simulink model "Ejercicio_2"  (R2013a)
settings: Solver=ode45  StartTime=0.0  StopTime=10.0  RelTol=1e-3
values from neighbouring files (symbols this model uses):
  G1 = 1/(s+7)    [Ecuaciones3_Practica_1.m]    (also in Ecuaciones_Practica_1.m; RLC_3.m = Vl/Vi; RL_1.m = w./sqrt(w.^2+(R/L)^2))
  G2 = 1/(s^2+2*s+3)    [Ecuaciones3_Practica_1.m]    (also in Ecuaciones_Practica_1.m; RLC_3.m = Vr/Vi; RL_1.m = (R/L)./sqrt(w.^2+(R/L)^2))
  G3 = 1/(s+4)    [Ecuaciones3_Practica_1.m]    (also in Ecuaciones_Practica_1.m)
  G4 = 1/s    [Ecuaciones3_Practica_1.m]    (also in Ecuaciones_Practica_1.m)
  G5 = 5/(s+7)    [Ecuaciones3_Practica_1.m]    (also in Ecuaciones_Practica_1.m)
  G6 = 1/(s^2+5*s+10)    [Ecuaciones3_Practica_1.m]    (also in Ecuaciones_Practica_1.m)
  G7 = 3/(s+2)    [Ecuaciones3_Practica_1.m]    (also in Ecuaciones_Practica_1.m)
  G8 = 1/(s+6)    [Ecuaciones3_Practica_1.m]    (also in Ecuaciones_Practica_1.m)
undefined symbols (not defined in the file or in its folder): Rs, Ys
settings Model: Creator=LuisFernando  LastModifiedBy=LuisFernando

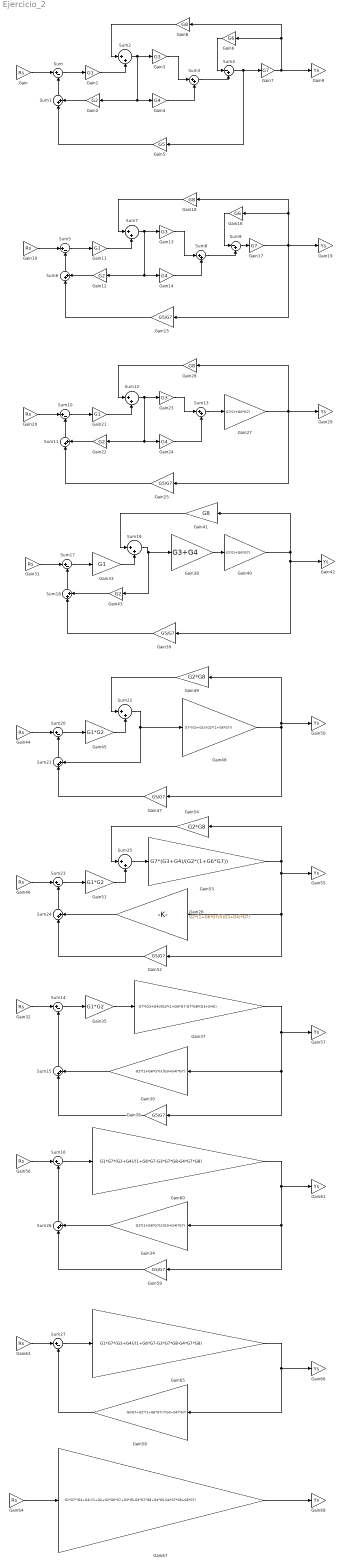
== system Ejercicio_2 ==
  Gain{,10,20,31..32,44,46,56,63..64} (10 alike) : Gain  Gain=Rs
  Gain{1,11,21,33} (4 alike) : Gain  Gain=G1
  Gain{2,12,22,43} (4 alike) : Gain  Gain=G2
  Gain13 : Gain  Gain=G3
  Gain14 : Gain  Gain=G4
  Gain{15,25,36,39,47,52,59} (7 alike) : Gain  Gain=G5/G7
  Gain16 : Gain  Gain=G6
  Gain17 : Gain  Gain=G7
  Gain{8,18,28,41} (4 alike) : Gain  Gain=G8
  Gain{9,19,29,42,50,55,57,61,66,68} (10 alike) : Gain  Gain=Ys
  Gain23 : Gain  Gain=G3
  Gain24 : Gain  Gain=G4
  Gain26 : Gain  Gain=G2*(1+G6*G7)/((G3+G4)*G7)
  Gain27 : Gain  Gain=G7/(1+G6*G7)
  Gain3 : Gain  Gain=G3
  Gain30 : Gain  Gain=G2*(1+G6*G7)/((G3+G4)*G7)
  Gain34 : Gain  Gain=G2*(1+G6*G7)/((G3+G4)*G7)
  Gain35 : Gain  Gain=G1*G2
  Gain37 : Gain  Gain=G7*(G3+G4)/(G2*(1+G6*G7-G7*G8*(G3+G4)))
  Gain38 : Gain  Gain=G3+G4
  Gain4 : Gain  Gain=G4
  Gain40 : Gain  Gain=G7/(1+G6*G7)
  Gain45 : Gain  Gain=G1*G2
  Gain48 : Gain  Gain=G7*(G3+G4)/(G2*(1+G6*G7))
  Gain49 : Gain  Gain=G2*G8
  Gain5 : Gain  Gain=G5
  Gain51 : Gain  Gain=G1*G2
  Gain53 : Gain  Gain=G7*(G3+G4)/(G2*(1+G6*G7))
  Gain54 : Gain  Gain=G2*G8
  Gain58 : Gain  Gain=G5/G7+G2*(1+G6*G7)/((G3+G4)*G7)
  Gain6 : Gain  Gain=G6
  Gain60 : Gain  Gain=G1*G7*(G3+G4)/(1+G6*G7-G3*G7*G8-G4*G7*G8)
  Gain65 : Gain  Gain=G1*G7*(G3+G4)/(1+G6*G7-G3*G7*G8-G4*G7*G8)
  Gain67 : Gain  Gain=G1*G7*(G3+G4)/(1+G2+G2*G6*G7+G3*G5-G3*G7*G8+G4*G5-G4*G7*G8+G6*G7)
  Gain7 : Gain  Gain=G7
  Sum{,5,10,14,16..17,20,23,27} (9 alike) : Sum  Inputs=|+-
  Sum{1..3,6..8,11..13,15,18..19,21..22,24..26} (17 alike) : Sum  Inputs=|++
  Sum4 : Sum  Inputs=|-+
  Sum9 : Sum  Inputs=|-+
  wires:
  Gain8/1 -> Sum2/1
  Gain1/1 -> Sum2/2
  Sum/1 -> Gain1/1
  Sum1/1 -> Sum/2
  Gain2/1 -> Sum1/2
  Gain5/1 -> Sum1/1
  Sum2/1 -> Gain4/1, Gain2/1, Gain3/1
  Gain3/1 -> Sum3/1
  Gain4/1 -> Sum3/2
  Sum3/1 -> Sum4/2
  Gain6/1 -> Sum4/1
  Sum4/1 -> Gain5/1, Gain7/1
  Gain7/1 -> Gain9/1, Gain8/1, Gain6/1
  Gain/1 -> Sum/1
  Gain18/1 -> Sum7/1
  Gain11/1 -> Sum7/2
  Sum5/1 -> Gain11/1
  Sum6/1 -> Sum5/2
  Gain12/1 -> Sum6/2
  Gain15/1 -> Sum6/1
  Sum7/1 -> Gain14/1, Gain12/1, Gain13/1
  Gain13/1 -> Sum8/1
  Gain14/1 -> Sum8/2
  Sum8/1 -> Sum9/2
  Gain16/1 -> Sum9/1
  Gain17/1 -> Gain15/1, Gain19/1, Gain18/1, Gain16/1
  Gain10/1 -> Sum5/1
  Sum9/1 -> Gain17/1
  Gain28/1 -> Sum12/1
  Gain21/1 -> Sum12/2
  Sum10/1 -> Gain21/1
  Sum11/1 -> Sum10/2
  Gain22/1 -> Sum11/2
  Gain25/1 -> Sum11/1
  Sum12/1 -> Gain24/1, Gain22/1, Gain23/1
  Gain23/1 -> Sum13/1
  Gain24/1 -> Sum13/2
  Gain27/1 -> Gain28/1, Gain25/1, Gain29/1
  Gain20/1 -> Sum10/1
  Sum13/1 -> Gain27/1
  Gain41/1 -> Sum19/1
  Gain33/1 -> Sum19/2
  Sum17/1 -> Gain33/1
  Sum18/1 -> Sum17/2
  Sum19/1 -> Gain43/1, Gain38/1
  Gain39/1 -> Sum18/1
  Gain40/1 -> Gain39/1, Gain42/1, Gain41/1
  Gain31/1 -> Sum17/1
  Gain38/1 -> Gain40/1
  Gain43/1 -> Sum18/2
  Gain49/1 -> Sum22/1
  Gain45/1 -> Sum22/2
  Sum20/1 -> Gain45/1
  Sum21/1 -> Sum20/2
  Gain47/1 -> Sum21/1
  Gain48/1 -> Gain50/1, Gain49/1, Gain47/1
  Gain44/1 -> Sum20/1
  Sum22/1 -> Sum21/2, Gain48/1
  Gain54/1 -> Sum25/1
  Gain51/1 -> Sum25/2
  Sum23/1 -> Gain51/1
  Sum24/1 -> Sum23/2
  Gain52/1 -> Sum24/1
  Gain53/1 -> Gain52/1, Gain26/1, Gain55/1, Gain54/1
  Gain46/1 -> Sum23/1
  Sum25/1 -> Gain53/1
  Gain26/1 -> Sum24/2
  Sum14/1 -> Gain35/1
  Sum15/1 -> Sum14/2
  Gain36/1 -> Sum15/1
  Gain37/1 -> Gain36/1, Gain30/1, Gain57/1
  Gain32/1 -> Sum14/1
  Gain30/1 -> Sum15/2
  Gain35/1 -> Gain37/1
  Sum26/1 -> Sum16/2
  Gain59/1 -> Sum26/1
  Gain60/1 -> Gain59/1, Gain34/1, Gain61/1
  Gain56/1 -> Sum16/1
  Gain34/1 -> Sum26/2
  Sum16/1 -> Gain60/1
  Gain65/1 -> Gain58/1, Gain66/1
  Gain63/1 -> Sum27/1
  Sum27/1 -> Gain65/1
  Gain58/1 -> Sum27/2
  Gain67/1 -> Gain68/1
  Gain64/1 -> Gain67/1
